simulink model "analog_emulators"  (R2020a)
settings: Solver=VariableStepAuto  StartTime=0.0  StopTime=tstop  RelTol=1e-3
libraries: cstblocks x2
settings Model: Creator=jambox  LastModifiedBy=jambox

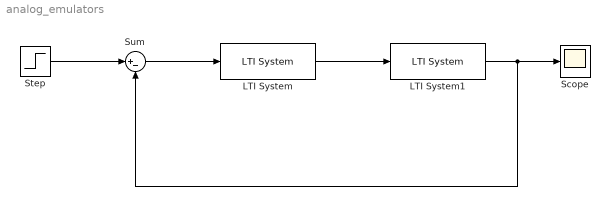
== system analog_emulators ==
  LTI System : cstblocks/LTI System  sys=D  IC=[]
  LTI System1 : cstblocks/LTI System  sys=P  IC=[]
  Scope : Scope
  Step : Step  SampleTime=0
  Sum : Sum  Inputs=|+-
  wires:
  Step/1 -> Sum/1
  Sum/1 -> LTI System/1
  LTI System/1 -> LTI System1/1
  LTI System1/1 -> Sum/2, Scope/1
